simulink model "test3_1_input"  (R2024a)
settings: Solver=VariableStepAuto  StartTime=0.0  StopTime=100  RelTol=1e-3
libraries: matrix_library x2
settings Model: Creator=katutu  LastModifiedBy=katutu

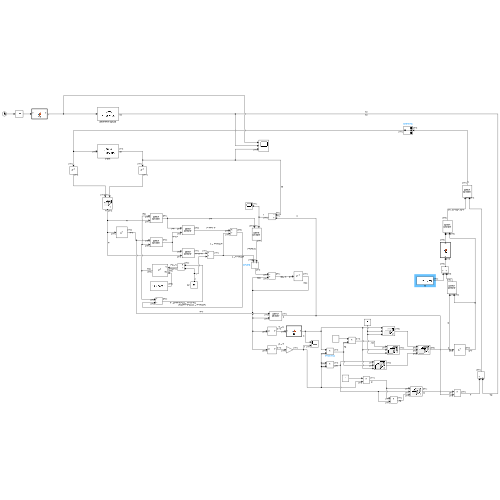
[thumbnail: Simulink's stored preview of the top-level diagram]
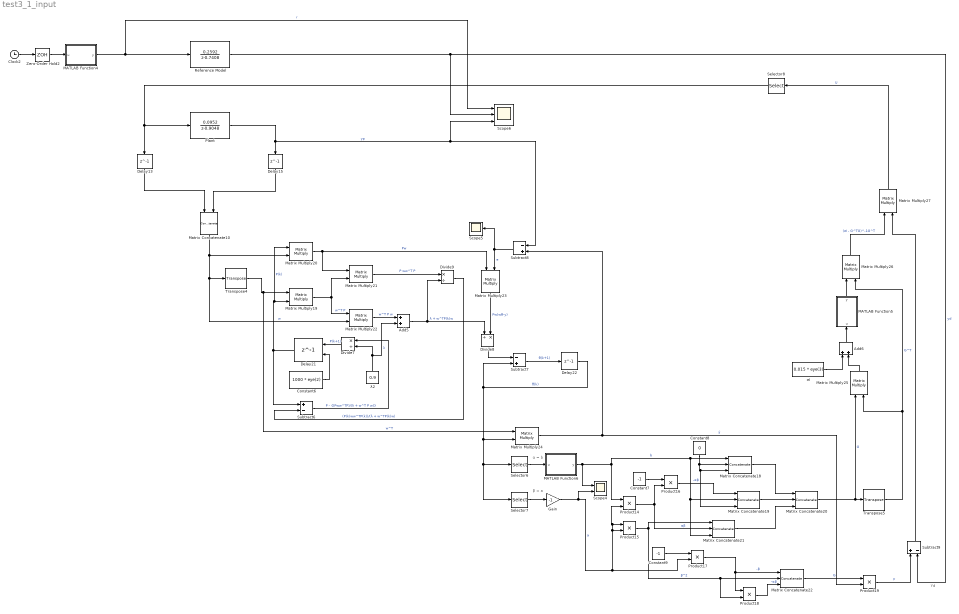
== system test3_1_input ==
  note: Yd
  note: α = b
  note: β = a
  Add5 : Sum
  Add6 : Sum
  Clock2 : Clock
  Constant6 : Constant  Value=1000 * eye(2)
  Constant7 : Constant  Value=-1
  Constant8 : Constant  Value=0
  Constant9 : Constant  Value=-1
  Delay13 : Delay  DelayLength=1  InitialCondition=0
  Delay15 : Delay  DelayLength=1  InitialCondition=0
  Delay21 : Delay  DelayLength=1  InitialConditionSource=Input port  InitialCondition=0
      settings: InputPortMap=u0,p4
  Delay22 : Delay  DelayLength=1  InitialCondition=[0 ; 0 ]
  Divide7 : Product  Inputs=*/
  Divide8 : Product  Inputs=/*
  Divide9 : Product  Inputs=*/
  Gain : Gain  Gain=-1
  MATLAB Function4 : MATLAB Function  TreatAsAtomicUnit=on
  MATLAB Function5 : MATLAB Function  TreatAsAtomicUnit=on
  MATLAB Function6 : MATLAB Function  TreatAsAtomicUnit=on
  Matrix Concatenate10 : Concatenate  Mode=Multidimensional array
  Matrix Concatenate18 : Concatenate  NumInputs=3  Mode=Multidimensional array  ConcatenateDimension=2
  Matrix Concatenate19 : Concatenate  NumInputs=3  Mode=Multidimensional array  ConcatenateDimension=2
  Matrix Concatenate20 : Concatenate  NumInputs=3  Mode=Multidimensional array
  Matrix Concatenate21 : Concatenate  NumInputs=3  Mode=Multidimensional array  ConcatenateDimension=2
  Matrix Concatenate22 : Concatenate  NumInputs=3  Mode=Multidimensional array
  Matrix Multiply{19..27} (9 alike) : Product  Multiplication=Matrix(*)
  Plant : DiscreteTransferFcn  Numerator=[0.0952]  Denominator=[1 -0.9048]
  Product{14..19} (6 alike) : Product
  Reference Model : DiscreteTransferFcn  Numerator=[0.2592]  Denominator=[1 -0.7408]
  Scope4 : Scope  NumInputPorts=2
  Scope5 : Scope
  Scope6 : Scope  NumInputPorts=3
  Selector6 : Selector  NumberOfDimensions=2  InputPortWidth=3  IndexOptions=Index vector (dialog),Index vector (dialog)  Indices=[1],1  OutputSizes=1,1
  Selector7 : Selector  NumberOfDimensions=2  InputPortWidth=3  IndexOptions=Index vector (dialog),Index vector (dialog)  Indices=[2],1  OutputSizes=1,1
  Selector8 : Selector  InputPortWidth=3  IndexOptions=Index vector (dialog)  Indices=[2]  OutputSizes=1
  Subtract6 : Sum  Inputs=+-
  Subtract7 : Sum  Inputs=-+
  Subtract8 : Sum  Inputs=-+
  Subtract9 : Sum  Inputs=+-
  Transpose4 : matrix_library/Transpose
  Transpose5 : matrix_library/Transpose
  Zero-Order Hold2 : ZeroOrderHold  SampleTime=-1
  λ2 : Constant  Value=0.9
  σI : Constant  Value=0.015 * eye(3)
  wires:
  Clock2/1 -> Zero-Order Hold2/1
  Zero-Order Hold2/1 -> MATLAB Function4/1(u)
  MATLAB Function4/1(y) -> Scope6/1, Reference Model/1  "r"
  Delay13/1 -> Matrix Concatenate10/1
  Delay15/1 -> Matrix Concatenate10/2
  Matrix Multiply19/1 -> Matrix Multiply22/1, Matrix Multiply21/2  "w^T P"
  Matrix Multiply21/1 -> Divide9/1  "P ww^T P"
  Matrix Multiply23/1 -> Divide8/2  "Pw(wθ-y)"
  Add5/1 -> Divide8/1, Divide9/2  "λ + w^TP(k)w"
  Constant6/1 -> Delay21/2
  Plant/1 -> Delay15/1, Subtract8/1, Scope6/3  "yp"
  Matrix Multiply22/1 -> Add5/1  "w^T P w"
  Delay21/1 -> Matrix Multiply19/2, Matrix Multiply20/1, Subtract6/1  "P(k)"
  Subtract7/1 -> Delay22/1  "θ(k+1)"
  Matrix Concatenate10/1 -> Transpose4/1, Matrix Multiply22/2, Matrix Multiply20/2  "w"
  Transpose4/1 -> Matrix Multiply24/1, Matrix Multiply19/1  "w^T"
  Subtract6/1 -> Divide7/1  "P - {(Pww^TP)/(λ + w^T P w)}"
  Matrix Multiply20/1 -> Matrix Multiply21/1, Matrix Multiply23/1  "Pw"
  λ2/1 -> Divide7/2, Add5/2  "λ"
  Delay22/1 -> Subtract7/2, Matrix Multiply24/2, Selector7/1, Selector6/1  "θ(k)"
  Divide9/1 -> Subtract6/2  "(P(k)ww^TP(k))/(λ + w^TP(k)w)"
  Divide7/1 -> Delay21/1  "P(k+1)"
  Divide8/1 -> Subtract7/1
  Matrix Multiply24/1 -> Product19/2, Subtract8/2  "ŷ"
  Subtract8/1 -> Matrix Multiply23/2, Scope5/1  "e"
  MATLAB Function6/1(y) -> Scope4/1, Matrix Concatenate21/3, Matrix Concatenate19/2, Matrix Concatenate18/1, Product14/1  "b"
  MATLAB Function5/1(y) -> Matrix Multiply26/1
  Constant8/1 -> Matrix Concatenate19/3, Matrix Concatenate18/3, Matrix Concatenate18/2
  Matrix Multiply25/1 -> Add6/2
  Add6/1 -> MATLAB Function5/1(u)
  Matrix Concatenate18/1 -> Matrix Concatenate20/1
  Matrix Concatenate20/1 -> Matrix Multiply25/1, Transpose5/1  "G"
  Matrix Multiply27/1 -> Selector8/1  "U"
  Product14/1 -> Matrix Concatenate21/2, Product16/2  "αβ"
  Matrix Concatenate21/1 -> Matrix Concatenate20/3
  Product16/1 -> Matrix Concatenate19/1  "-αβ"
  σI/1 -> Add6/1
  Subtract9/1 -> Matrix Multiply27/2
  Transpose5/1 -> Matrix Multiply25/2, Matrix Multiply26/2  "G^T"
  Matrix Multiply26/1 -> Matrix Multiply27/1  "(σI - G^TG)^-1G^T"
  Constant7/1 -> Product16/1
  Matrix Concatenate19/1 -> Matrix Concatenate20/2
  Product15/1 -> Matrix Concatenate21/1, Product18/2, Matrix Concatenate22/2  "β^2"
  Constant9/1 -> Product17/1
  Product17/1 -> Product18/1, Matrix Concatenate22/1  "-β"
  Product18/1 -> Matrix Concatenate22/3  "-αβ"
  Matrix Concatenate22/1 -> Product19/1  "G"
  Product19/1 -> Subtract9/1  "F"
  Reference Model/1 -> Subtract9/2, Scope6/2  "yd"
  Selector7/1 -> Gain/1
  Selector6/1 -> MATLAB Function6/1(u)
  Gain/1 -> Scope4/2, Product14/2, Product15/1, Product15/2, Product17/2  "a"
  Selector8/1 -> Delay13/1, Plant/1

== matlab function test3_1_input/MATLAB Function5 ==
  data: u input; y output
function y = fcn(u)

y = inv(u);

== matlab function test3_1_input/MATLAB Function6 ==
  data: u input; y output
function y = fcn(u)

e = 0.01;

if(u == 0)
    y = e;

elseif(abs(u) < 0.01)
    y = e * sign(u);
else
    y = u;
end

== matlab function test3_1_input/MATLAB Function4 ==
  data: u input; y output
function y = fcn(u)

if(u<50)
    y=1;
else
    y=-1;
end
